simulink model "hardware_sim_two_topology"  (R2023b)
settings: Solver=VariableStepAuto  StartTime=0.0  StopTime=0.1  MaxStep=1e-6  RelTol=1e-3
libraries: spsSeriesRLCBranchLib x18, spsVoltageMeasurementLib x18, spsCurrentMeasurementLib x16, spsDiodeLib x13, spsACVoltageSourceLib x6, spsMeanLib x4, spsMosfetLib x3, spsDCVoltageSourceLib x2, spsGroundLib x2, spspowerguiLib x2
settings Model: Creator=elife  LastModifiedBy=elife
settings SolverCC: ZeroCrossAlgorithm=Adaptive
settings DataIOCC: ReturnWorkspaceOutputs=off
settings DebuggingCC: IgnoredZcDiagnostic=none

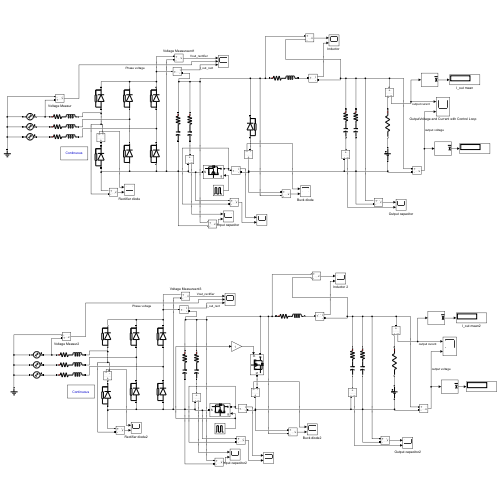
[thumbnail: Simulink's stored preview of the top-level diagram]
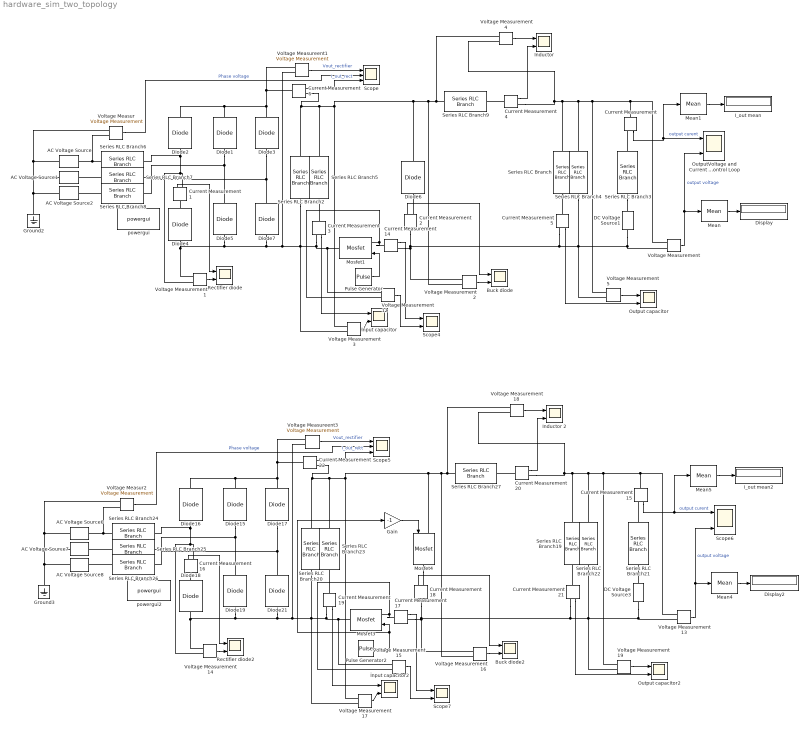
== system hardware_sim_two_topology ==
  AC Voltage Source : spsACVoltageSourceLib/AC Voltage Source  Amplitude=25*sqrt(2)/sqrt(3)  Phase=0  Frequency=50  SampleTime=0  Measurements=None  BusType=swing  Pref=10e3  Qref=0  Qmin=-inf  Qmax=+inf
  AC Voltage Source1 : spsACVoltageSourceLib/AC Voltage Source  Amplitude=25*sqrt(2)/sqrt(3)  Phase=120  Frequency=50  SampleTime=0  Measurements=None  BusType=swing  Pref=10e3  Qref=0  Qmin=-inf  Qmax=+inf
  AC Voltage Source2 : spsACVoltageSourceLib/AC Voltage Source  Amplitude=25*sqrt(2)/sqrt(3)  Phase=240  Frequency=50  SampleTime=0  Measurements=None  BusType=swing  Pref=10e3  Qref=0  Qmin=-inf  Qmax=+inf
  AC Voltage Source6 : spsACVoltageSourceLib/AC Voltage Source  Amplitude=25*sqrt(2)/sqrt(3)  Phase=0  Frequency=50  SampleTime=0  Measurements=None  BusType=swing  Pref=10e3  Qref=0  Qmin=-inf  Qmax=+inf
  AC Voltage Source7 : spsACVoltageSourceLib/AC Voltage Source  Amplitude=25*sqrt(2)/sqrt(3)  Phase=120  Frequency=50  SampleTime=0  Measurements=None  BusType=swing  Pref=10e3  Qref=0  Qmin=-inf  Qmax=+inf
  AC Voltage Source8 : spsACVoltageSourceLib/AC Voltage Source  Amplitude=25*sqrt(2)/sqrt(3)  Phase=240  Frequency=50  SampleTime=0  Measurements=None  BusType=swing  Pref=10e3  Qref=0  Qmin=-inf  Qmax=+inf
  Buck diode : Scope  NumInputPorts=2
  Buck diode2 : Scope  NumInputPorts=2
  Current Measurement{,1..6,14..22} (16 alike) : spsCurrentMeasurementLib/Current Measurement  PhasorSimulation=off  OutputType=Complex  PSBequivalent=0
  DC Voltage Source1 : spsDCVoltageSourceLib/DC Voltage Source  Amplitude=12  Measurements=None
  DC Voltage Source3 : spsDCVoltageSourceLib/DC Voltage Source  Amplitude=12  Measurements=None
  Diode{1..5,7,15..19,21} (12 alike) : spsDiodeLib/Diode  Ron=0.013  Lon=0  Vf=0.7  IC=0  UseSnubber=0  Rs=1.5  Cs=1.7e-7  Measurements=off
  Diode6 : spsDiodeLib/Diode  Ron=0.013  Lon=0  Vf=0.7  IC=0  UseSnubber=0  Rs=2.4  Cs=7.7e-8  Measurements=off
  Display : Display
  Display2 : Display
  Gain : Gain  Gain=-1
  Ground2 : spsGroundLib/Ground  LConnTagsString=a
  Ground3 : spsGroundLib/Ground  LConnTagsString=a
  I_out mean : Display
  I_out mean2 : Display
  "Inductor " : Scope  NumInputPorts=2
  Inductor 2 : Scope  NumInputPorts=2
  Mean{,1,4..5} (4 alike) : spsMeanLib/Mean  Freq=60  Vinit=0  Ts=0
  Mosfet1 : spsMosfetLib/Mosfet  Ron=0.013  Lon=0  Rd=0.013  Vfd=0.7  IC=0  Rs=2  Cs=1.7e-7  Measurements=off
  Mosfet3 : spsMosfetLib/Mosfet  Ron=0.013  Lon=0  Rd=0.013  Vfd=0.7  IC=0  Rs=2  Cs=1.7e-7  Measurements=off
  Mosfet4 : spsMosfetLib/Mosfet  Ron=0.013  Lon=0  Rd=0.013  Vfd=0.7  IC=0  Rs=2.4  Cs=7.7e-7  Measurements=off
  Output capacitor : Scope  NumInputPorts=2
  Output capacitor2 : Scope  NumInputPorts=2
  OutputVoltage and Current with Control Loop : Scope  NumInputPorts=2
  Pulse Generator : DiscretePulseGenerator  PulseType=Time based  Period=1/10000  PulseWidth=39.4
  Pulse Generator2 : DiscretePulseGenerator  PulseType=Time based  Period=1/10000  PulseWidth=39.4
  Rectifier diode : Scope  NumInputPorts=2
  Rectifier diode2 : Scope  NumInputPorts=2
  Scope : Scope  NumInputPorts=3
  Scope4 : Scope  NumInputPorts=2
  Scope5 : Scope  NumInputPorts=3
  Scope6 : Scope  NumInputPorts=2
  Scope7 : Scope  NumInputPorts=2
  Series RLC Branch{,4,19,22} (4 alike) : spsSeriesRLCBranchLib/Series RLC Branch  LConnTagsString=__new0  RConnTagsString=__new0  BranchType=RC  Resistance=0.08  Inductance=1e-3  SetiL0=off  InitialCurrent=0  Capacitance=470e-6  Setx0=off  InitialVoltage=0  Measurements=None
  Series RLC Branch{2,5,20,23} (4 alike) : spsSeriesRLCBranchLib/Series RLC Branch  LConnTagsString=__new0  RConnTagsString=__new0  BranchType=RC  Resistance=0.08  Inductance=1e-3  SetiL0=off  InitialCurrent=0  Capacitance=680e-6  Setx0=off  InitialVoltage=0  Measurements=None
  Series RLC Branch21 : spsSeriesRLCBranchLib/Series RLC Branch  LConnTagsString=__new0  RConnTagsString=__new0  BranchType=R  Resistance=20e-3  Inductance=1e-3  SetiL0=off  InitialCurrent=0  Capacitance=680e-6  Setx0=off  InitialVoltage=0  Measurements=None
  Series RLC Branch{6..8,24..26} (6 alike) : spsSeriesRLCBranchLib/Series RLC Branch  LConnTagsString=__new0  RConnTagsString=__new0  BranchType=RL  Resistance=5e-6  Inductance=1e-4  SetiL0=off  InitialCurrent=0  Capacitance=1e-6  Setx0=off  InitialVoltage=0  Measurements=None
  Series RLC Branch27 : spsSeriesRLCBranchLib/Series RLC Branch  LConnTagsString=__new0  RConnTagsString=__new0  BranchType=RL  Resistance=5e-3  Inductance=680e-6  SetiL0=off  InitialCurrent=0  Capacitance=1e-6  Setx0=off  InitialVoltage=0  Measurements=None
  Series RLC Branch3 : spsSeriesRLCBranchLib/Series RLC Branch  LConnTagsString=__new0  RConnTagsString=__new0  BranchType=R  Resistance=20e-3  Inductance=1e-3  SetiL0=off  InitialCurrent=0  Capacitance=680e-6  Setx0=off  InitialVoltage=0  Measurements=None
  Series RLC Branch9 : spsSeriesRLCBranchLib/Series RLC Branch  LConnTagsString=__new0  RConnTagsString=__new0  BranchType=RL  Resistance=5e-3  Inductance=680e-6  SetiL0=off  InitialCurrent=0  Capacitance=1e-6  Setx0=off  InitialVoltage=0  Measurements=None
  Voltage Measur : spsVoltageMeasurementLib/Voltage Measurement  PhasorSimulation=off  OutputType=Complex  PSBequivalent=0
  Voltage Measur2 : spsVoltageMeasurementLib/Voltage Measurement  PhasorSimulation=off  OutputType=Complex  PSBequivalent=0
  Voltage Measureent1 : spsVoltageMeasurementLib/Voltage Measurement  PhasorSimulation=off  OutputType=Complex  PSBequivalent=0
  Voltage Measureent3 : spsVoltageMeasurementLib/Voltage Measurement  PhasorSimulation=off  OutputType=Complex  PSBequivalent=0
  Voltage Measurement{,1..5,12..19} (14 alike) : spsVoltageMeasurementLib/Voltage Measurement  PhasorSimulation=off  OutputType=Complex  PSBequivalent=0
  powergui : spspowerguiLib/powergui  Priority=1  SimulationMode=Continuous  SampleTime=50e-6  frequency=60  Iterations=50  frequencyindice=50  Pbase=100e6  ErrMax=1e-4  UnitsV=kV  UnitsW=MW  buscounter=0  FunctionMessages=off  echomessages=off  EnableUseOfTLC=off  CurrentSourceSwitches=off  DisableSnubberDevices=off  DisableRonSwitches=off  DisableVfSwitches=off  DisplayEquations=off  AutomaticDiscreteSolvers=off  SolverType=Tustin/Backward Euler (TBE)  Interpol=off  ExternalGateDelay=off  methode=off  Ts=100  x0status=blocks  SPID=on  SwTol=0  HookPort=off  NonlinearTolerance=1e-4  nMaxIteration=100  ContinueOnMaxIteration=off  RestoreLinks=warning  ResistiveCurrentMeasurement=off  Frange=[0:2:500]  Ylog=off  Xlog=on  ShowGrid=off  save=off  variable=ZData  structure=0  ZoomFFT=off  StartTime=0.0  cycles=1  DisplayStyle=1  fundamental=60  FreqAxis=off  MaxFrequency=1000  frequencyindicesteady=1  RmsSteady=1  display=off
  powergui2 : spspowerguiLib/powergui  Priority=1  SimulationMode=Continuous  SampleTime=50e-6  frequency=60  Iterations=50  frequencyindice=50  Pbase=100e6  ErrMax=1e-4  UnitsV=kV  UnitsW=MW  buscounter=0  FunctionMessages=off  echomessages=off  EnableUseOfTLC=off  CurrentSourceSwitches=off  DisableSnubberDevices=off  DisableRonSwitches=off  DisableVfSwitches=off  DisplayEquations=off  AutomaticDiscreteSolvers=off  SolverType=Tustin/Backward Euler (TBE)  Interpol=off  ExternalGateDelay=off  methode=off  Ts=100  x0status=blocks  SPID=on  SwTol=0  HookPort=off  NonlinearTolerance=1e-4  nMaxIteration=100  ContinueOnMaxIteration=off  RestoreLinks=warning  ResistiveCurrentMeasurement=off  Frange=[0:2:500]  Ylog=off  Xlog=on  ShowGrid=off  save=off  variable=ZData  structure=0  ZoomFFT=off  StartTime=0.0  cycles=1  DisplayStyle=1  fundamental=60  FreqAxis=off  MaxFrequency=1000  frequencyindicesteady=1  RmsSteady=1  display=off
  İnput capacitor : Scope  NumInputPorts=2
  İnput capacitor2 : Scope  NumInputPorts=2
  wires:
  Voltage Measurement/1 -> OutputVoltage and Current with Control Loop/2, Mean/1  "output voltage"
  Mean/1 -> Display/1
  Voltage Measureent1/1 -> Scope/1  "Vout_rectifier"
  Voltage Measur/1 -> Scope/2  "Phase voltage"
  Mean1/1 -> I_out mean/1
  Current Measurement1/1 -> Rectifier diode/1
  Current Measurement2/1 -> Buck diode/1
  Voltage Measurement2/1 -> Buck diode/2
  Current Measurement3/1 -> İnput capacitor/1
  Current Measurement4/1 -> "Inductor "/2
  Voltage Measurement4/1 -> "Inductor "/1
  Current Measurement5/1 -> Output capacitor/2
  Voltage Measurement5/1 -> Output capacitor/1
  Voltage Measurement3/1 -> İnput capacitor/2
  Voltage Measurement1/1 -> Rectifier diode/2
  Current Measurement6/1 -> Scope/3  "I_out_rect"
  Current Measurement14/1 -> Scope4/1
  Voltage Measurement12/1 -> Scope4/2
  Voltage Measurement13/1 -> Scope6/2, Mean4/1  "output voltage"
  Voltage Measurement19/1 -> Output capacitor2/1
  Current Measurement22/1 -> Scope5/3  "I_out_rect"
  Mean5/1 -> I_out mean2/1
  Voltage Measurement18/1 -> Inductor 2/1
  Current Measurement21/1 -> Output capacitor2/2
  Mean4/1 -> Display2/1
  Current Measurement16/1 -> Rectifier diode2/1
  Current Measurement19/1 -> İnput capacitor2/1
  Current Measurement18/1 -> Buck diode2/1
  Voltage Measurement16/1 -> Buck diode2/2
  Current Measurement20/1 -> Inductor 2/2
  Voltage Measureent3/1 -> Scope5/1  "Vout_rectifier"
  Current Measurement15/1 -> Mean5/1, Scope6/1  "output curent"
  Voltage Measurement15/1 -> Scope7/2
  Voltage Measurement14/1 -> Rectifier diode2/2
  Voltage Measur2/1 -> Scope5/2  "Phase voltage"
  Voltage Measurement17/1 -> İnput capacitor2/2
  Current Measurement17/1 -> Scope7/1
  Pulse Generator2/1 -> Gain/1, Mosfet3/1
  Gain/1 -> Mosfet4/1
  Current Measurement/1 -> Mean1/1, OutputVoltage and Current with Control Loop/1  "output curent"
  Pulse Generator/1 -> Mosfet1/1
  connections:
  AC Voltage Source2/LConn1 -- Ground2/LConn1 -- Voltage Measur/LConn2 -- AC Voltage Source/LConn1 -- AC Voltage Source1/LConn1
  Voltage Measurement/LConn1 -- Voltage Measurement5/LConn1 -- Current Measurement4/RConn1 -- Voltage Measurement4/LConn2 -- Series RLC Branch/LConn1 -- Series RLC Branch4/LConn1 -- Current Measurement/LConn1
  Series RLC Branch3/LConn1 -- Current Measurement/RConn1
  Series RLC Branch6/RConn1 -- Voltage Measurement1/LConn2 -- Current Measurement1/RConn1 -- Diode2/LConn1
  Series RLC Branch7/RConn1 -- Diode5/RConn1 -- Diode1/LConn1
  Series RLC Branch8/RConn1 -- Diode7/RConn1 -- Diode3/LConn1
  Series RLC Branch3/RConn1 -- DC Voltage Source1/RConn1
  Mosfet1/RConn1 -- Voltage Measurement12/LConn1 -- Current Measurement3/RConn1 -- Voltage Measurement3/LConn2 -- Diode7/LConn1 -- Voltage Measurement1/LConn1 -- Diode4/LConn1 -- Diode5/LConn1 -- Voltage Measureent1/LConn2 -- Series RLC Branch2/RConn1
  Series RLC Branch6/LConn1 -- AC Voltage Source/RConn1 -- Voltage Measur/LConn1
  Series RLC Branch7/LConn1 -- AC Voltage Source1/RConn1
  Series RLC Branch8/LConn1 -- AC Voltage Source2/RConn1
  Current Measurement4/LConn1 -- Series RLC Branch9/RConn1
  Diode2/RConn1 -- Diode1/RConn1 -- Current Measurement6/LConn1 -- Voltage Measureent1/LConn1 -- Diode3/RConn1
  Voltage Measurement5/LConn2 -- DC Voltage Source1/LConn1 -- Voltage Measurement/LConn2 -- Series RLC Branch4/RConn1 -- Current Measurement5/RConn1 -- Current Measurement2/LConn1 -- Voltage Measurement2/LConn1 -- Current Measurement14/RConn1
  Current Measurement1/LConn1 -- Diode4/RConn1
  Current Measurement2/RConn1 -- Diode6/LConn1
  Current Measurement3/LConn1 -- Series RLC Branch5/RConn1
  Current Measurement5/LConn1 -- Series RLC Branch/RConn1
  Voltage Measurement2/LConn2 -- Voltage Measurement3/LConn1 -- Current Measurement6/RConn1 -- Series RLC Branch2/LConn1 -- Series RLC Branch5/LConn1 -- Diode6/RConn1 -- Voltage Measurement4/LConn1 -- Series RLC Branch9/LConn1
  Current Measurement14/LConn1 -- Voltage Measurement12/LConn2 -- Mosfet1/LConn1
  Current Measurement17/RConn1 -- Voltage Measurement16/LConn1 -- Current Measurement18/LConn1 -- Voltage Measurement19/LConn2 -- DC Voltage Source3/LConn1 -- Voltage Measurement13/LConn2 -- Series RLC Branch22/RConn1 -- Current Measurement21/RConn1
  Series RLC Branch22/LConn1 -- Current Measurement20/RConn1 -- Voltage Measurement18/LConn2 -- Series RLC Branch19/LConn1 -- Voltage Measurement13/LConn1 -- Current Measurement15/LConn1 -- Voltage Measurement19/LConn1
  Voltage Measureent3/LConn1 -- Diode16/RConn1 -- Diode15/RConn1 -- Diode17/RConn1 -- Current Measurement22/LConn1
  Diode17/LConn1 -- Series RLC Branch26/RConn1 -- Diode21/RConn1
  Series RLC Branch23/LConn1 -- Current Measurement22/RConn1 -- Series RLC Branch20/LConn1 -- Voltage Measurement16/LConn2 -- Voltage Measurement18/LConn1 -- Series RLC Branch27/LConn1 -- Mosfet4/LConn1 -- Voltage Measurement17/LConn1
  Series RLC Branch20/RConn1 -- Voltage Measurement17/LConn2 -- Diode21/LConn1 -- Voltage Measurement14/LConn1 -- Diode18/LConn1 -- Diode19/LConn1 -- Voltage Measureent3/LConn2 -- Mosfet3/RConn1 -- Voltage Measurement15/LConn1 -- Current Measurement19/RConn1
  Current Measurement16/RConn1 -- Series RLC Branch24/RConn1 -- Diode16/LConn1 -- Voltage Measurement14/LConn2
  AC Voltage Source6/LConn1 -- AC Voltage Source8/LConn1 -- Ground3/LConn1 -- AC Voltage Source7/LConn1 -- Voltage Measur2/LConn2
  Diode15/LConn1 -- Series RLC Branch25/RConn1 -- Diode19/RConn1
  Mosfet3/LConn1 -- Current Measurement17/LConn1 -- Voltage Measurement15/LConn2
  Voltage Measur2/LConn1 -- Series RLC Branch24/LConn1 -- AC Voltage Source6/RConn1
  Series RLC Branch21/LConn1 -- Current Measurement15/RConn1
  Current Measurement19/LConn1 -- Series RLC Branch23/RConn1
  Current Measurement21/LConn1 -- Series RLC Branch19/RConn1
  Series RLC Branch26/LConn1 -- AC Voltage Source8/RConn1
  Current Measurement16/LConn1 -- Diode18/RConn1
  Series RLC Branch21/RConn1 -- DC Voltage Source3/RConn1
  Current Measurement20/LConn1 -- Series RLC Branch27/RConn1
  Series RLC Branch25/LConn1 -- AC Voltage Source7/RConn1
  Mosfet4/RConn1 -- Current Measurement18/RConn1
